simulink model "simulation"  (R2021b)
settings: Solver=ode3  StartTime=0.0  StopTime=0.2  FixedStep=Ts  RelTol=1e-3
model workspace (MAT data in the model file):
  J_x = 8e-06
  J_y = 7.85e-06
  K0_x = 0.1
  K0_y = 0.1
  Kf_x = 0.00565
  Kf_y = 0.00553
  Ki_x = 0.00424
  Ki_y = 0.00406
  Kp_x = -0.1074
  Kp_y = -0.1545
  Kr_x = 1
  Kr_y = 1
  Kt_x = -931
  Kt_y = -914
  SNR = 1
  Ts = 1e-06
  aire_photodiode = 7.02
  angle_range = 15
  angle_x = 0
  angle_z = 0
  barcode_image = [92 38 38 38 38 38 38 38 38 38 38 38 ... (1616960 elements, 1304x1240)]
  fc_highpass = 300
  fc_transimpedance = 10000
  fini_surface = 0
  gain_filtre = 100
  gain_photodiode = 0.42
  gain_transimpedance = 1500000
  hauteur = 35
  largeur = 70
  lum_elec = 0.001
  lum_nat = 0.001
  noyau_gaussien = [0 0 0 0 0 0 0 0 0 0 0 0 ... (2601 elements, 51x51)]
  p_x = 0
  p_y = 0
  p_z = -100
  puissance_laser = 1
  pwm_freq = 30000
  pwm_period = 3e-05
  ratio_x = 0.0806451612903
  ratio_y = 0.0766871165644
  rayon = 0
  scan_freq = 15
  scan_period = 0.1
  seuil_comparateur = 1
  temps_echantillonnage = 5
  tolerance_decodage = 0.01
  v_range = 0.261799387799
libraries: simulink x5
(part 2 of 2)

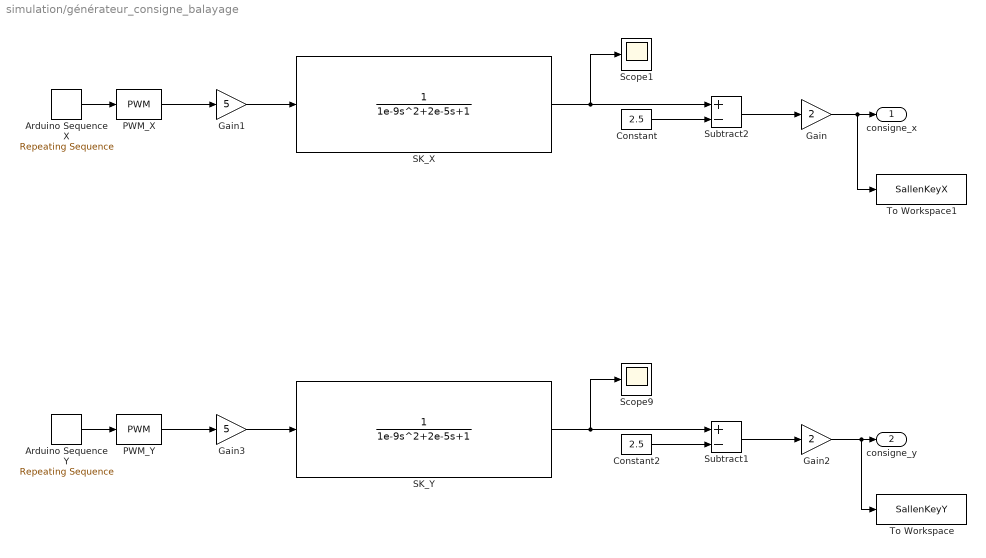
== system simulation/générateur_consigne_balayage ==
  Arduino Sequence X : simulink/Sources/Repeating Sequence  rep_seq_t=[0 1/(2*scan_freq) 1/scan_freq 1/scan_freq+1e-6 1/scan_freq+1/(2*scan_freq) 1/scan_freq+1/scan_freq]  rep_seq_y=[0.5-v_range 0.5+v_range 0.5-v_range 0.5 0.5 0.5]
  Arduino Sequence Y : simulink/Sources/Repeating Sequence  rep_seq_t=[0 1/(2*scan_freq) 1/scan_freq 1/scan_freq+1e-6 1/scan_freq+1/(2*scan_freq) 1/scan_freq+1/scan_freq]  rep_seq_y=[0.5 0.5 0.5 0.5-v_range 0.5+v_range 0.5-v_range]
  Constant : Constant  Value=2.5
  Constant2 : Constant  Value=2.5
  Gain : Gain  Gain=2
  Gain1 : Gain  Gain=5
  Gain2 : Gain  Gain=2
  Gain3 : Gain  Gain=5
  PWM_X : simulink/Discontinuities/PWM  DisableCoverage=on  Period=pwm_period  DisallowZeroDutyCycle=off  RunAtFixedTimeIntervals=on  SampleTime=Ts
  PWM_Y : simulink/Discontinuities/PWM  DisableCoverage=on  Period=pwm_period  DisallowZeroDutyCycle=off  RunAtFixedTimeIntervals=on  SampleTime=Ts
  SK_X : TransferFcn  Denominator=[1e-9 2e-5 1]
  SK_Y : TransferFcn  Denominator=[1e-9 2e-5 1]
  Scope1 : Scope
  Scope9 : Scope
  Subtract1 : Sum  Inputs=+-
  Subtract2 : Sum  Inputs=+-
  To Workspace : ToWorkspace  VariableName=SallenKeyY  SaveFormat=Timeseries  SampleTime=-1
  To Workspace1 : ToWorkspace  VariableName=SallenKeyX  SaveFormat=Timeseries  SampleTime=-1
  consigne_x : Outport
  consigne_y : Outport  Port=2
  wires:
  Gain/1 -> To Workspace1/1, consigne_x/1
  Constant2/1 -> Subtract1/2
  Arduino Sequence Y/1 -> PWM_Y/1
  PWM_X/1 -> Gain1/1
  Subtract1/1 -> Gain2/1
  Subtract2/1 -> Gain/1
  PWM_Y/1 -> Gain3/1
  Gain1/1 -> SK_X/1
  SK_Y/1 -> Scope9/1, Subtract1/1
  Gain2/1 -> To Workspace/1, consigne_y/1
  Arduino Sequence X/1 -> PWM_X/1
  Constant/1 -> Subtract2/2
  Gain3/1 -> SK_Y/1
  SK_X/1 -> Scope1/1, Subtract2/1

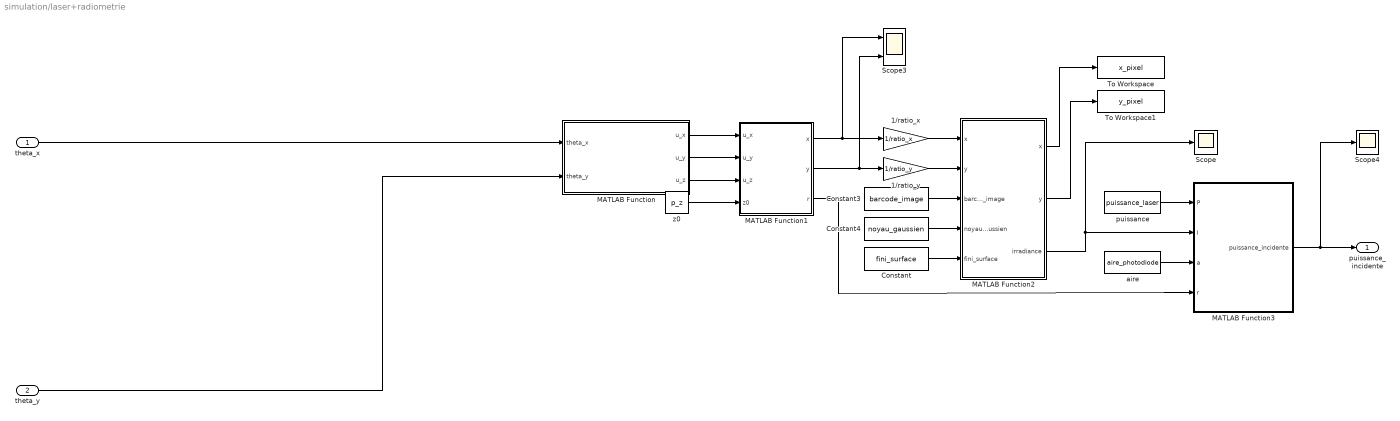
== system simulation/laser+radiometrie ==
  theta_x : Inport
  theta_y : Inport  Port=2
  1/ratio_x : Gain  Gain=1/ratio_x
  1/ratio_y : Gain  Gain=1/ratio_y
  Constant : Constant  Value=fini_surface
  Constant3 : Constant  Value=barcode_image
  Constant4 : Constant  Value=noyau_gaussien
  MATLAB Function : MATLAB Function  TreatAsAtomicUnit=on
  MATLAB Function1 : MATLAB Function  TreatAsAtomicUnit=on
  MATLAB Function2 : MATLAB Function  TreatAsAtomicUnit=on
  MATLAB Function3 : MATLAB Function  TreatAsAtomicUnit=on
  Scope : Scope
  Scope3 : Scope  NumInputPorts=2
  Scope4 : Scope
  To Workspace : ToWorkspace  VariableName=x_pixel  SaveFormat=Timeseries  SampleTime=-1
  To Workspace1 : ToWorkspace  VariableName=y_pixel  SaveFormat=Timeseries  SampleTime=-1
  aire : Constant  Value=aire_photodiode
  puissance : Constant  Value=puissance_laser
  z0 : Constant  Value=p_z
  puissance_incidente : Outport
  wires:
  MATLAB Function2/2(y) -> To Workspace1/1
  aire/1 -> MATLAB Function3/3(a)
  theta_x/1 -> MATLAB Function/1(theta_x)
  Constant4/1 -> MATLAB Function2/4(noyau_gaussien)
  theta_y/1 -> MATLAB Function/2(theta_y)
  Constant3/1 -> MATLAB Function2/3(barcode_image)
  MATLAB Function/2(u_y) -> MATLAB Function1/2(u_y)
  MATLAB Function2/3(irradiance) -> Scope/1, MATLAB Function3/2(I)
  z0/1 -> MATLAB Function1/4(z0)
  1/ratio_x/1 -> MATLAB Function2/1("x ")
  MATLAB Function1/1(x) -> 1/ratio_x/1, Scope3/1
  MATLAB Function2/1(x) -> To Workspace/1
  MATLAB Function/3(u_z) -> MATLAB Function1/3(u_z)
  MATLAB Function1/3(r) -> MATLAB Function3/4(r)
  MATLAB Function1/2(y) -> 1/ratio_y/1, Scope3/2
  MATLAB Function/1(u_x) -> MATLAB Function1/1(u_x)
  1/ratio_y/1 -> MATLAB Function2/2("y ")
  MATLAB Function3/1(puissance_incidente) -> Scope4/1, puissance_incidente/1
  puissance/1 -> MATLAB Function3/1(P)
  Constant/1 -> MATLAB Function2/5(fini_surface)

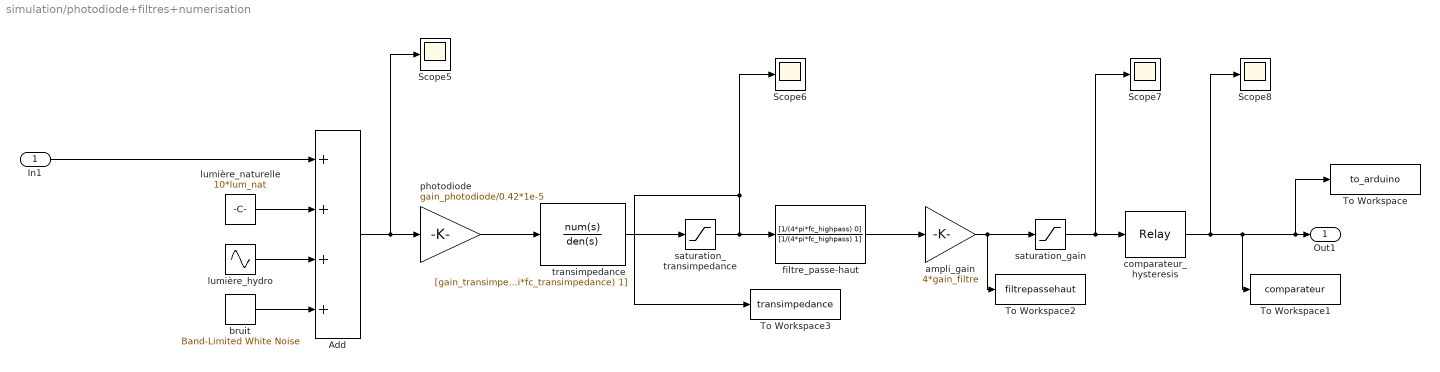
== system simulation/photodiode+filtres+numerisation ==
  In1 : Inport
  Add : Sum  Inputs=++++
  Scope{5..8} (4 alike) : Scope
  To Workspace : ToWorkspace  VariableName=to_arduino  SaveFormat=Timeseries  SampleTime=Ts*temps_echantillonnage
  To Workspace1 : ToWorkspace  VariableName=comparateur  SaveFormat=Timeseries  SampleTime=-1
  To Workspace2 : ToWorkspace  VariableName=filtrepassehaut  SaveFormat=Timeseries  SampleTime=-1
  To Workspace3 : ToWorkspace  VariableName=transimpedance  SaveFormat=Timeseries  SampleTime=-1
  ampli_gain : Gain  Gain=4*gain_filtre
  bruit : simulink/Sources/Band-Limited White Noise  Cov=[SNR*1e-17]  Ts=Ts  seed=[23341]
  comparateur_hysteresis : Relay  OnSwitchValue=seuil_comparateur  OffSwitchValue=-seuil_comparateur  OnOutputValue=5
  filtre_passe-haut : TransferFcn  Numerator=[1/(4*pi*fc_highpass) 0]  Denominator=[1/(4*pi*fc_highpass) 1]
  lumière_hydro : Sin  Amplitude=0.01*lum_elec  Frequency=240*pi  SampleTime=Ts
  lumière_naturelle : Constant  Value=10*lum_nat
  photodiode : Gain  Gain=gain_photodiode/0.42*1e-5
  saturation_gain : Saturate  UpperLimit=5  LowerLimit=-5
  saturation_transimpedance : Saturate  UpperLimit=5  LowerLimit=-5
  transimpedance : TransferFcn  Numerator=[gain_transimpedance]  Denominator=[1/(2*pi*fc_transimpedance) 1]
  Out1 : Outport
  wires:
  In1/1 -> Add/1
  bruit/1 -> Add/4
  ampli_gain/1 -> To Workspace2/1, saturation_gain/1
  lumière_naturelle/1 -> Add/2
  saturation_gain/1 -> Scope7/1, comparateur_hysteresis/1
  transimpedance/1 -> saturation_transimpedance/1
  lumière_hydro/1 -> Add/3
  filtre_passe-haut/1 -> ampli_gain/1
  Add/1 -> Scope5/1, photodiode/1
  comparateur_hysteresis/1 -> To Workspace1/1, To Workspace/1, Out1/1, Scope8/1
  photodiode/1 -> transimpedance/1
  saturation_transimpedance/1 -> To Workspace3/1, Scope6/1, filtre_passe-haut/1

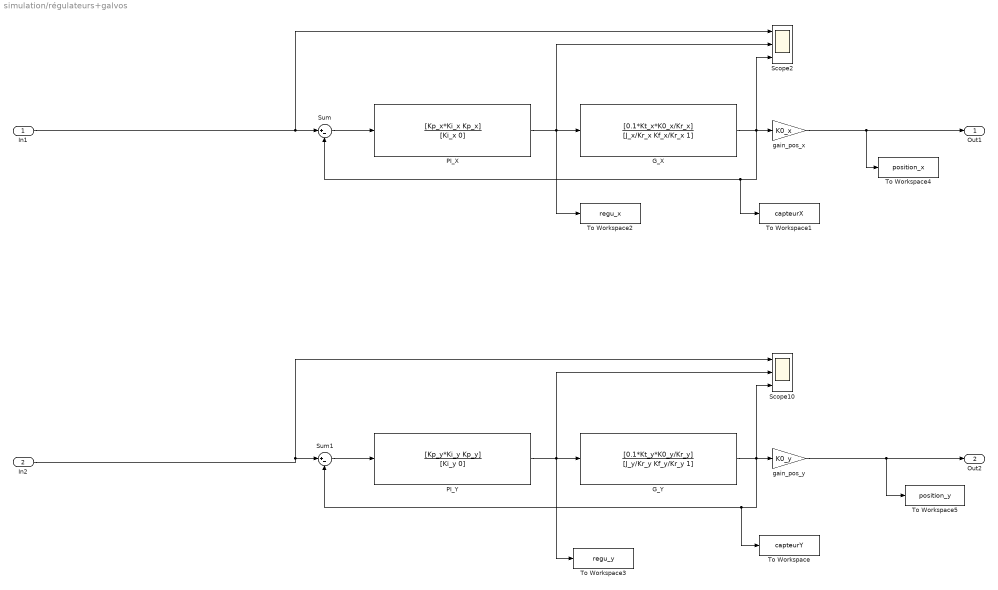
== system simulation/régulateurs+galvos ==
  In1 : Inport
  In2 : Inport  Port=2
  G_X : TransferFcn  Numerator=[0.1*Kt_x*K0_x/Kr_x]  Denominator=[J_x/Kr_x Kf_x/Kr_x 1]
  G_Y : TransferFcn  Numerator=[0.1*Kt_y*K0_y/Kr_y]  Denominator=[J_y/Kr_y Kf_y/Kr_y 1]
  PI_X : TransferFcn  Numerator=[Kp_x*Ki_x Kp_x]  Denominator=[Ki_x 0]
  PI_Y : TransferFcn  Numerator=[Kp_y*Ki_y Kp_y]  Denominator=[Ki_y 0]
  Scope10 : Scope  NumInputPorts=3
  Scope2 : Scope  NumInputPorts=3
  Sum : Sum  Inputs=|+-
  Sum1 : Sum  Inputs=|+-
  To Workspace : ToWorkspace  VariableName=capteurY  SaveFormat=Timeseries  SampleTime=-1
  To Workspace1 : ToWorkspace  VariableName=capteurX  SaveFormat=Timeseries  SampleTime=-1
  To Workspace2 : ToWorkspace  VariableName=regu_x  SaveFormat=Timeseries  SampleTime=-1
  To Workspace3 : ToWorkspace  VariableName=regu_y  SaveFormat=Timeseries  SampleTime=-1
  To Workspace4 : ToWorkspace  VariableName=position_x  SaveFormat=Timeseries  SampleTime=-1
  To Workspace5 : ToWorkspace  VariableName=position_y  SaveFormat=Timeseries  SampleTime=-1
  gain_pos_x : Gain  Gain=K0_x
  gain_pos_y : Gain  Gain=K0_y
  Out1 : Outport
  Out2 : Outport  Port=2
  wires:
  Sum1/1 -> PI_Y/1
  In2/1 -> Scope10/1, Sum1/1
  G_Y/1 -> To Workspace/1, Sum1/2, gain_pos_y/1, Scope10/3
  PI_Y/1 -> Scope10/2, To Workspace3/1, G_Y/1
  G_X/1 -> To Workspace1/1, Sum/2, gain_pos_x/1, Scope2/3
  Sum/1 -> PI_X/1
  In1/1 -> Scope2/1, Sum/1
  PI_X/1 -> To Workspace2/1, Scope2/2, G_X/1
  gain_pos_x/1 -> To Workspace4/1, Out1/1
  gain_pos_y/1 -> To Workspace5/1, Out2/1

== matlab function simulation/laser+radiometrie/MATLAB Function1 ==
  data: x output; u_x input; y output; u_y input; u_z input; z0 input; r output
function [x,y,r] = intersection(u_x, u_y, u_z, z0)
    % intersection laser-code_barre
    % ratio [mm/pixel]
    t = z0 / u_z;
    x = t*u_x;
    y = t*u_y;
    r = sqrt(z0^2);
end

== matlab function simulation/laser+radiometrie/MATLAB Function ==
  data: theta_x input; u_x output; theta_y input; u_y output; u_z output
function [u_x, u_y, u_z] = reflexion_laser(theta_x, theta_y)
    % reflexion matrix (snell's vectorial law)
    u_x = 1 - 2*cos(theta_x - pi/4)^2;
    u_y = (1 - 2*sin(theta_y + pi/4)^2)*(-2*cos(theta_x - pi/4)*sin(theta_x - pi/4));
    u_z = 4*cos(theta_y + pi/4)*sin(theta_y + pi/4)*cos(theta_x - pi/4)*sin(theta_x - pi/4);
    % vector_laser
    u = [u_x, u_y, u_z];
    u = u/norm(u);
    u_x = u(1); u_y = u(2); u_z = u(3);
end

== matlab function simulation/laser+radiometrie/MATLAB Function2 ==
  data: x output; y output; x input; irradiance output; y input; barcode_image input; noyau_gaussien input; fini_surface input
function [x,y,irradiance] = convolution(x,y,barcode_image,noyau_gaussien,fini_surface)
%CONVOLUTION
    i_size = size(barcode_image);
    n = i_size(1); m = i_size(2);
    y = fix(y + n/2); x = fix(x + m/2);

    k_size = size(noyau_gaussien);
    p = k_size(1); o = k_size(2);
    b = fix(p/2); a = fix(o/2);
    
    if (x > a) && (x < m-a) && (y > b) && (y < n-b) %   convolution
        irradiance = sum(im2double(barcode_image(y-b:y+b,x-a:x+a)).*noyau_gaussien,'all');
    else
        irradiance = 1;
    end
    irradiance = irradiance + fini_surface;
end

== matlab function simulation/laser+radiometrie/MATLAB Function3 ==
  data: P input; I input; puissance_incidente output; a input; r input
function puissance_incidente  = puissance(P, I, a, r)
    % PUISSANCE
    % Integral on solid angle (small approximation)
    puissance_incidente = P*I*a/r^2;
end
